simulink model "controller_arduino"  (R2023b)
settings: Solver=FixedStepDiscrete  StartTime=0.0  StopTime=inf  FixedStep=0.1  RelTol=1e-3  EnableMultiTasking=on
libraries: arduinolib x11, simulink x4, hdlsllib x2
settings Model: ExtModeTrigDuration=2  Creator=DAUIN-Win10  LastModifiedBy=Matteo
settings OptimizationCC: EnhancedBackFolding=on  PassReuseOutputArgsAs=Individual arguments  ZeroExternalMemoryAtStartup=off  ZeroInternalMemoryAtStartup=off  MaxStackSize=64  OptimizeBlockOrder=speed  DifferentSizesBufferReuse=on  OptimizationCustomize=off  EfficientTunableParamExpr=on
settings DebuggingCC: ParameterTunabilityLossMsg=error  UnconnectedInputMsg=warning  UnconnectedOutputMsg=warning  UnconnectedLineMsg=warning  ModelReferenceSymbolNameMessage=none
settings HardwareCC: ProdBitPerInt=16  ProdBitPerPointer=16  ProdBitPerSizeT=16  ProdBitPerPtrDiffT=16  ProdLargestAtomicFloat=None  ProdWordSize=8  ProdHWDeviceType=Atmel->AVR
settings ModelReferenceCC: EnableRefExpFcnMdlSchedulingChecks=on
settings SFSimCC: MATLABDynamicMemAlloc=off
settings RTWCC: Description=Embedded Coder  SystemTargetFile=ert.tlc  HardwareBoard=Arduino Uno  TemplateMakefile=ert_default_tmf  Toolchain=Arduino AVR  BuildConfiguration=Faster Runs  DLArmComputeVersion=19.05
settings CodeAppCC: ForceParamTrailComments=on  IgnoreCustomStorageClasses=off  OperatorAnnotations=on  SimulinkDataObjDesc=on  SFDataObjDesc=on  InsertBlockDesc=on
settings ERTTargetCC: SupportContinuousTime=on  SupportVariableSizeSignals=on  ExtModeTransport=3  ExtModeStaticAlloc=on  ExtModeAutomaticAllocSize=off  ExtModeStaticAllocSize=250  ExtModeMexFile=ext_xcp  ExtModeIntrfLevel=Level2 - Open

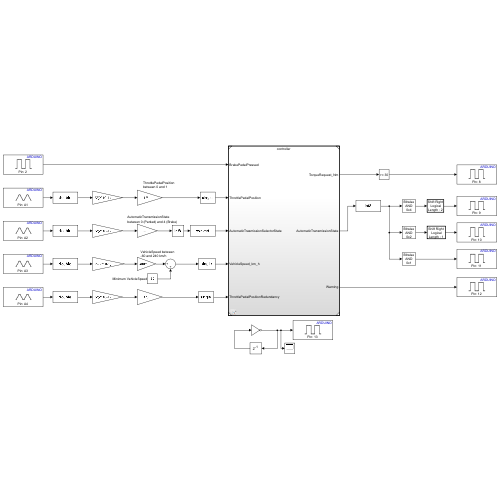
[thumbnail: Simulink's stored preview of the top-level diagram]
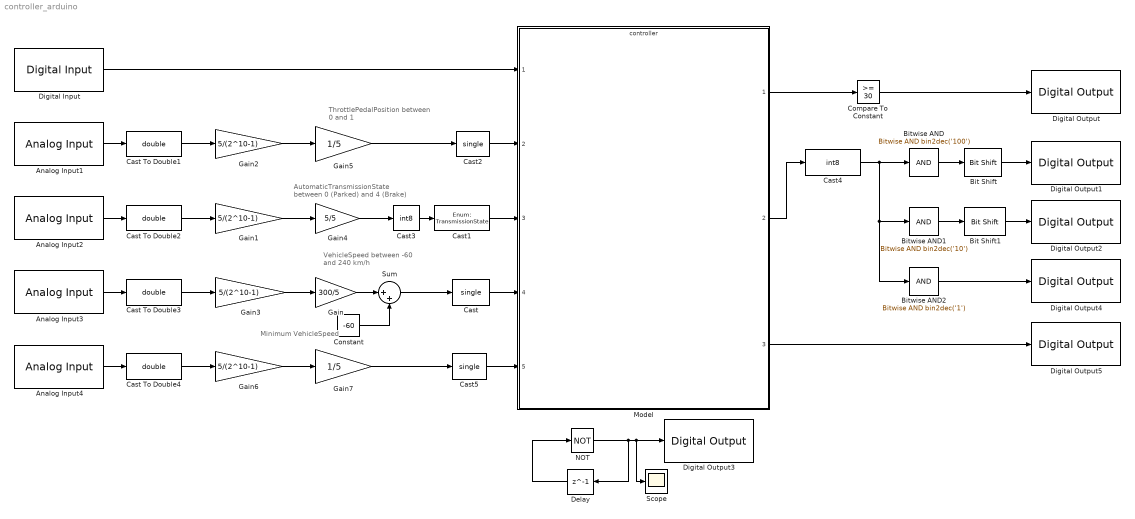
== system controller_arduino ==
  note: ThrottlePedalPosition
      | between 0 and 1
  note: Minimum VehicleSpeed
  note: AutomaticTransmissionState
      | between 0 (Parked) and 4 (Brake)
  note: VehicleSpeed between
      | -60 and 240 km/h
  Analog Input1 : arduinolib/Analog Input  pinNumber=1  ReadResultsOnly=off  ConversionTriggerSource=Software  ExternalTriggerType=uint32( 0 )  OutputDataType=uint16  EnableConversionCompleteNotify=off  EnableOuputStatus=off  SampleTime=-1  blockPlatform=arduino
  Analog Input2 : arduinolib/Analog Input  pinNumber=2  ReadResultsOnly=off  ConversionTriggerSource=Software  ExternalTriggerType=uint32( 0 )  OutputDataType=uint16  EnableConversionCompleteNotify=off  EnableOuputStatus=off  SampleTime=-1  blockPlatform=arduino
  Analog Input3 : arduinolib/Analog Input  pinNumber=3  ReadResultsOnly=off  ConversionTriggerSource=Software  ExternalTriggerType=uint32( 0 )  OutputDataType=uint16  EnableConversionCompleteNotify=off  EnableOuputStatus=off  SampleTime=-1  blockPlatform=arduino
  Analog Input4 : arduinolib/Analog Input  pinNumber=4  ReadResultsOnly=off  ConversionTriggerSource=Software  ExternalTriggerType=uint32( 0 )  OutputDataType=uint16  EnableConversionCompleteNotify=off  EnableOuputStatus=off  SampleTime=-1  blockPlatform=arduino
  Bit Shift : hdlsllib/Logic and Bit Operations/Bit Shift  mode=Shift Right Logical  N=2
  Bit Shift1 : hdlsllib/Logic and Bit Operations/Bit Shift  mode=Shift Right Logical  N=1
  Bitwise AND : simulink/Logic and Bit Operations/Bitwise Operator  logicop=AND  UseBitMask=on  BitMask=bin2dec('100')  BitMaskRealWorld=Stored Integer
      settings: LibrarySourceBlock=|
      | simulink/Quick Insert/Logic and Bit
      | Operations/Bitwise AND
  Bitwise AND1 : simulink/Logic and Bit Operations/Bitwise Operator  logicop=AND  UseBitMask=on  BitMask=bin2dec('10')  BitMaskRealWorld=Stored Integer
      settings: LibrarySourceBlock=|
      | simulink/Quick Insert/Logic and Bit
      | Operations/Bitwise AND
  Bitwise AND2 : simulink/Logic and Bit Operations/Bitwise Operator  logicop=AND  UseBitMask=on  BitMask=bin2dec('1')  BitMaskRealWorld=Stored Integer
      settings: LibrarySourceBlock=|
      | simulink/Quick Insert/Logic and Bit
      | Operations/Bitwise AND
  Cast : DataTypeConversion  OutDataTypeStr=single  SaturateOnIntegerOverflow=off  RndMeth=Floor
  Cast To Double{1..4} (4 alike) : DataTypeConversion  OutDataTypeStr=double  SaturateOnIntegerOverflow=off  RndMeth=Floor
  Cast1 : DataTypeConversion  OutDataTypeStr=Enum: TransmissionState  SaturateOnIntegerOverflow=off  RndMeth=Floor
  Cast2 : DataTypeConversion  OutDataTypeStr=single  SaturateOnIntegerOverflow=off  RndMeth=Floor
  Cast3 : DataTypeConversion  OutDataTypeStr=int8  SaturateOnIntegerOverflow=off  RndMeth=Floor
  Cast4 : DataTypeConversion  OutDataTypeStr=int8  SaturateOnIntegerOverflow=off  RndMeth=Floor
  Cast5 : DataTypeConversion  OutDataTypeStr=single  SaturateOnIntegerOverflow=off  RndMeth=Floor
  Compare To Constant : simulink/Logic and Bit Operations/Compare To Constant  relop=>=  const=30  OutDataTypeStr=uint8
  Constant : Constant  Value=-60
  Delay : Delay  DelayLength=1  SampleTime=0.5
  Digital Input : arduinolib/Digital Input  pinNumber=2  mode=Default  Direction=input  SampleTime=0.1  blockPlatform=arduino
  Digital Output : arduinolib/Digital Output  pinNumber=8  Direction=output  blockPlatform=arduino
  Digital Output1 : arduinolib/Digital Output  pinNumber=9  Direction=output  blockPlatform=arduino
  Digital Output2 : arduinolib/Digital Output  pinNumber=10  Direction=output  blockPlatform=arduino
  Digital Output3 : arduinolib/Digital Output  pinNumber=13  Direction=output  blockPlatform=arduino
  Digital Output4 : arduinolib/Digital Output  pinNumber=11  Direction=output  blockPlatform=arduino
  Digital Output5 : arduinolib/Digital Output  pinNumber=12  Direction=output  blockPlatform=arduino
  Gain : Gain  Gain=300/5
  Gain{1..3,6} (4 alike) : Gain  Gain=5/(2^10-1)
  Gain4 : Gain  Gain=5/5
  Gain5 : Gain  Gain=1/5
  Gain7 : Gain  Gain=1/5
  Model : ModelReference  ModelNameDialog=controller  SimulationMode=Normal  ModelReferenceVersion=5.8
  NOT : Logic  Operator=NOT  IconShape=distinctive  AllPortsSameDT=off  OutDataTypeStr=boolean
  Scope : Scope
  Sum : Sum  Inputs=|++
  wires:
  Analog Input1/1 -> Cast To Double1/1
  NOT/1 -> Delay/1, Scope/1, Digital Output3/1
  Delay/1 -> NOT/1
  Analog Input3/1 -> Cast To Double3/1
  Analog Input2/1 -> Cast To Double2/1
  Cast To Double1/1 -> Gain2/1
  Cast To Double2/1 -> Gain1/1
  Cast To Double3/1 -> Gain3/1
  Gain2/1 -> Gain5/1
  Digital Input/1 -> Model/1
  Gain3/1 -> Gain/1
  Gain/1 -> Sum/1
  Constant/1 -> Sum/2
  Gain1/1 -> Gain4/1
  Cast/1 -> Model/4
  Sum/1 -> Cast/1
  Cast1/1 -> Model/3
  Cast2/1 -> Model/2
  Gain5/1 -> Cast2/1
  Compare To Constant/1 -> Digital Output/1
  Model/1 -> Compare To Constant/1
  Bit Shift/1 -> Digital Output1/1
  Bitwise AND/1 -> Bit Shift/1
  Bit Shift1/1 -> Digital Output2/1
  Cast3/1 -> Cast1/1
  Gain4/1 -> Cast3/1
  Model/2 -> Cast4/1
  Cast4/1 -> Bitwise AND2/1, Bitwise AND1/1, Bitwise AND/1
  Bitwise AND1/1 -> Bit Shift1/1
  Bitwise AND2/1 -> Digital Output4/1
  Model/3 -> Digital Output5/1
  Gain6/1 -> Gain7/1
  Gain7/1 -> Cast5/1
  Analog Input4/1 -> Cast To Double4/1
  Cast5/1 -> Model/5
  Cast To Double4/1 -> Gain6/1
